simulink model "simulink_motorDC"  (R2017a)
settings: Solver=ode45  StartTime=0.0  StopTime=60  MaxStep=0.005  RelTol=1e-3  EnableMultiTasking=on
InitFcn:
  | % Intervalo de amostragem
  | T = 0.05;
values from neighbouring files (symbols this model uses):
  b = 0.1    [script_motorDC.m]
  den = [325 -600 275]    [script_motorDC.m]
  J = 0.01    [script_motorDC.m]
  K = 0.01    [script_motorDC.m]
  L = 0.5    [script_motorDC.m]
  num = [21600 -39960 18468]    [script_motorDC.m]
  R = 1    [script_motorDC.m]
  ts = 0.05*4/10    (= 0.02)    [script_motorDC.m]
undefined symbols (not defined in the file or in its folder): sigbuilder_block
settings Model: Creator=torres  LastModifiedBy=Italo
settings DataIOCC: LimitDataPoints=on  SaveFormat=Array
settings OptimizationCC: ExpressionDepthLimit=2147483647  LifeSpan=inf
settings DebuggingCC: UnderspecifiedInitializationDetection=Classic  MergeDetectMultiDrivingBlocksExec=none  SolverPrmCheckMsg=warning  FcnCallInpInsideContextMsg=warning  StateNameClashWarn=warning  SFUnexpectedBacktrackingDiag=warning  SFNoUnconditionalDefaultTransitionDiag=warning  SFExecutionAtInitializationDiag=none
settings HardwareCC: ProdBitPerPointer=32  ProdBitPerSizeT=32  ProdBitPerPtrDiffT=32  ProdLargestAtomicFloat=None  ProdIntDivRoundTo=Undefined  ProdEndianess=Unspecified  ProdWordSize=32  ProdHWDeviceType=32-bit Generic
settings ModelReferenceCC: PropagateSignalLabelsOutOfModel=off
settings GRTTargetCC: TargetLangStandard=C89/C90 (ANSI)  CombineOutputUpdateFcns=off  GRTInterface=on
settings ConfigComp: CovMetricSettings=dw  CovHtmlReporting=on  CovSaveCumulativeToWorkspaceVar=on  CovSaveSingleToWorkspaceVar=on  CovExternalEMLEnable=off

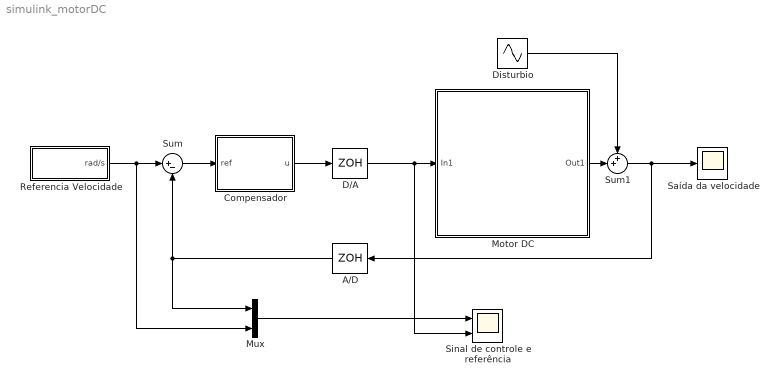
== system simulink_motorDC ==
  A/D : ZeroOrderHold  SampleTime=ts
  Compensador : Subsystem
  D/A : ZeroOrderHold  SampleTime=ts
  Disturbio : Sin  Amplitude=5  Frequency=0.1  SampleTime=0
  Motor DC : Subsystem
      mask Display: image(imread('images.jpeg'))
  Mux : Mux  Inputs=2
  Referencia Velocidade : Subsystem  Tag=STV Subsys  LoadFcn=sigbuilder_block('load');  StartFcn=sigbuilder_block('start');  StopFcn=sigbuilder_block('stop');  ClipboardFcn=sigbuilder_block('clipboard');  mask(Sigbuilder block){tuvar=[0:10]}
      mask help: Sigbuilder GUI
      mask init:
      | if ~strcmp(get_param(bdroot(gcbh),'SimulationStatus'),'stopped') tuvar = sigbuilder_block('maskInit'); end
      settings: CopyFcn=sigbuilder_block('copy');  DeleteFcn=sigbuilder_block('delete');  ModelCloseFcn=sigbuilder_block('modelClose');  PreSaveFcn=sigbuilder_block('preSave');  PauseFcn=sigbuilder_block('pause')  ContinueFcn=sigbuilder_block('continue')  NameChangeFcn=sigbuilder_block('namechange');  OpenFcn=sigbuilder_block('open',[212 137.6 876 383.2 ]);  CloseFcn=sigbuilder_block('close');
      mask Display: plot(0, 0, 100, 100,[2, 2, 32, 32, 2], [68, 8, 8, 68, 68],[32, 2], [38, 38], [32, 19, 2],[53, 60, 44], [32, 17, 17, 2],[16, 16, 31, 31]);txt = getActiveGroup(gcbh);text(2, 100, txt,'verticalAlignment', 'top');
  Saída da velocidade : Scope
  Sinal de controle e referência : Scope  NumInputPorts=2
  Sum : Sum  Inputs=|+-
  Sum1 : Sum  Inputs=++|
  wires:
  Referencia Velocidade/1(rad/s) -> Mux/2, Sum/1
  D/A/1 -> Sinal de controle e referência/2, Motor DC/1(In1)
  A/D/1 -> Sum/2, Mux/1
  Mux/1 -> Sinal de controle e referência/1
  Disturbio/1 -> Sum1/1
  Motor DC/1(Out1) -> Sum1/2
  Sum/1 -> Compensador/1(ref)
  Compensador/1(u) -> D/A/1
  Sum1/1 -> Saída da velocidade/1, A/D/1

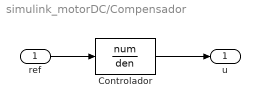
== system simulink_motorDC/Compensador ==
  ref : Inport
  Controlador : DiscreteTransferFcn  Numerator=num  Denominator=den
  u : Outport
  wires:
  ref/1 -> Controlador/1
  Controlador/1 -> u/1

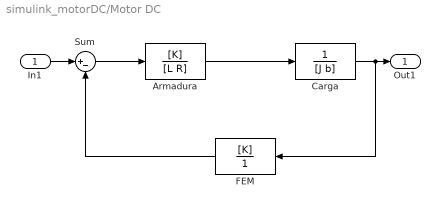
== system simulink_motorDC/Motor DC ==
  In1 : Inport
  Armadura : TransferFcn  Numerator=[K]  Denominator=[L R]  ContinuousStateAttributes='torque'
  Carga : TransferFcn  Denominator=[J b]  ContinuousStateAttributes='velocidade'
  FEM : TransferFcn  Numerator=[K]  Denominator=1
  Sum : Sum  Inputs=|+-
  Out1 : Outport
  wires:
  Armadura/1 -> Carga/1
  Sum/1 -> Armadura/1
  FEM/1 -> Sum/2
  Carga/1 -> FEM/1, Out1/1
  In1/1 -> Sum/1

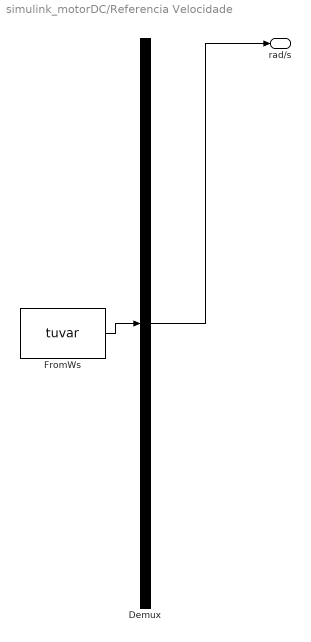
== system simulink_motorDC/Referencia Velocidade ==
  Demux : Demux  Tag=STV Demux  Outputs=1
  FromWs : FromWorkspace  Tag=STV FromWs  VariableName=tuvar  SampleTime=0
      SigBuilderData=|
      | common.afterFinalStr = 'Extrapolate'
      | common.sampleTime = 0
      | dataSet.timeRange = [0 60]
      | dataSet.name = 'Group 1'
      | sbobj.Groups.Name = 'Group 1'
      | sbobj.Groups.Signals.Name = 'rad/s'
      | sbobj.Groups.Signals.XData = [0 10 30 40 60]
      | sbobj.Groups.Signals.YData = [0 100 100 0 0]
      | sbobj.Groups.TimeRange = [0 60]
  rad/s : Outport  Tag=STV Outport
  wires:
  Demux/1 -> rad/s/1
  FromWs/1 -> Demux/1
